simulink model "PID_LOOP"  (R2024b)
settings: Solver=FixedStepAuto  StartTime=0.0  StopTime=60  RelTol=1e-3
model workspace (MAT data in the model file):
  Drag_Constants = 1
  mass = [5.51 5.51 5.51 1 1 1]
  mass_6a = [5 5 5 1 1 1]
values from neighbouring files (symbols this model uses):
  drag_wrench = [ ... (first row only)    [constants.m]    (also in constants.mat = [0.41 0 0 0 0 0 0 0.5 0 0 0 0 ... (36 elements, 6x6)])
  g = 9.8067    [constants.m]    (also in constants.mat = 9.80665)
  I_x = 1    [constants.mat]
  I_y = 1    [constants.mat]
  I_z = 1    [constants.mat]
  m = mc + mp    (= 6)    [calculate_inertia.m]    (also in constants.mat = 5.51; mass_properties.mat = 10)
  volume = 0.0074    [constants.m]    (also in constants.mat = 0.0073741788)
  volume_center = [0, 0, -0.07]    [constants.m]    (also in constants.mat = [0 0 0.1])
  water_density = 997    [constants.m]    (also in constants.mat = 1000)
  wrench = eval(w)    [calculate_wrench.m]    (also in constants.m = geometry_properties.wrench; constants.mat = [0 0 0 0 -0.7071 -0.7071 -0.7071 -0.7071 0 0 0 0 ... (48 ele; geometry_properties.mat = [0 0 -1 0.22 0.25 0 0 0 -1 -0.22 0.25 0 ... (48 elements, 6x; wrench.m)
undefined symbols (not defined in the file or in its folder): pwm_stop
libraries: slpidlib x6, simulink x3, shareduavrstlib x1
settings Model: Creator=zenyn  LastModifiedBy=Pamarit - Test
settings DataIOCC: LoggingToFile=on
settings OptimizationCC: DefaultParameterBehavior=Inlined  UseDivisionForNetSlopeComputation=on  GainParamInheritBuiltInType=on  UseFloatMulNetSlope=on  DefaultUnderspecifiedDataType=single  InlineInvariantSignals=on  ReuseModelBlockBuffer=off  PassReuseOutputArgsAs=Individual arguments  ZeroExternalMemoryAtStartup=off  ZeroInternalMemoryAtStartup=off  NoFixptDivByZeroProtection=on  EfficientFloat2IntCast=on  LifeSpan=1  OptimizeDataStoreBuffers=off  BusAssignmentInplaceUpdate=off  EfficientTunableParamExpr=on
settings DebuggingCC: ParameterTunabilityLossMsg=error  SFUnexpectedBacktrackingDiag=warning  SFNoUnconditionalDefaultTransitionDiag=warning  UnderSpecifiedDimensionMsg=warning
settings HardwareCC: ProdLongLongMode=on
settings SFSimCC: MATLABDynamicMemAlloc=off
settings RTWCC: Description=Embedded Coder  SystemTargetFile=ert.tlc  TemplateMakefile=ert_default_tmf  GenerateReport=on  Toolchain=MinGW64 | gmake (64-bit Windows)  BuildConfiguration=Debug  IncludeHyperlinkInReport=on  LaunchReport=on  TargetLang=C++  GenerateTraceInfo=on  GenerateTraceReport=on  GenerateTraceReportSl=on  GenerateTraceReportSf=on  GenerateTraceReportEml=on
settings CodeAppCC: ForceParamTrailComments=on  IgnoreCustomStorageClasses=off  OperatorAnnotations=on  SimulinkDataObjDesc=on  SFDataObjDesc=on  CustomSymbolStrGlobalVar=rt$N$M  CustomSymbolStrType=$N$M  CustomSymbolStrFcn=$N$M$F  CustomSymbolStrMacro=$N$M  InsertBlockDesc=on  EnableCustomComments=on  ReqsInCode=on
settings ERTTargetCC: TargetLangStandard=C++11 (ISO)  GenerateSampleERTMain=on  IncludeMdlTerminateFcn=off  CombineSignalStateStructs=on  SupportAbsoluteTime=off  CodeInterfacePackaging=C++ class  SupportComplex=off  SupportContinuousTime=on  SupportNonInlinedSFcns=on  RootIOFormat=Structure reference  ERTCustomFileTemplate=example_file_process.tlc  ERTFilePackagingFormat=CompactWithDataFile  ConvertIfToSwitch=off

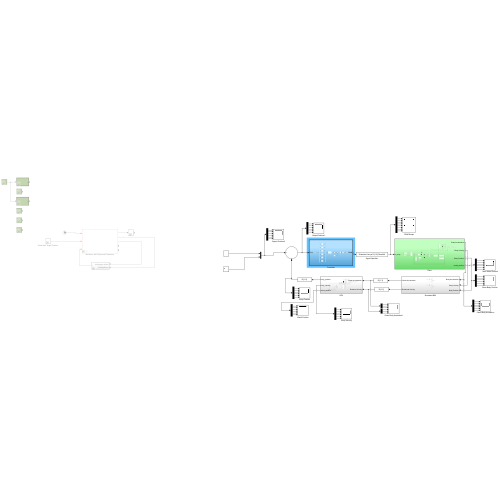
[thumbnail: Simulink's stored preview of the top-level diagram]
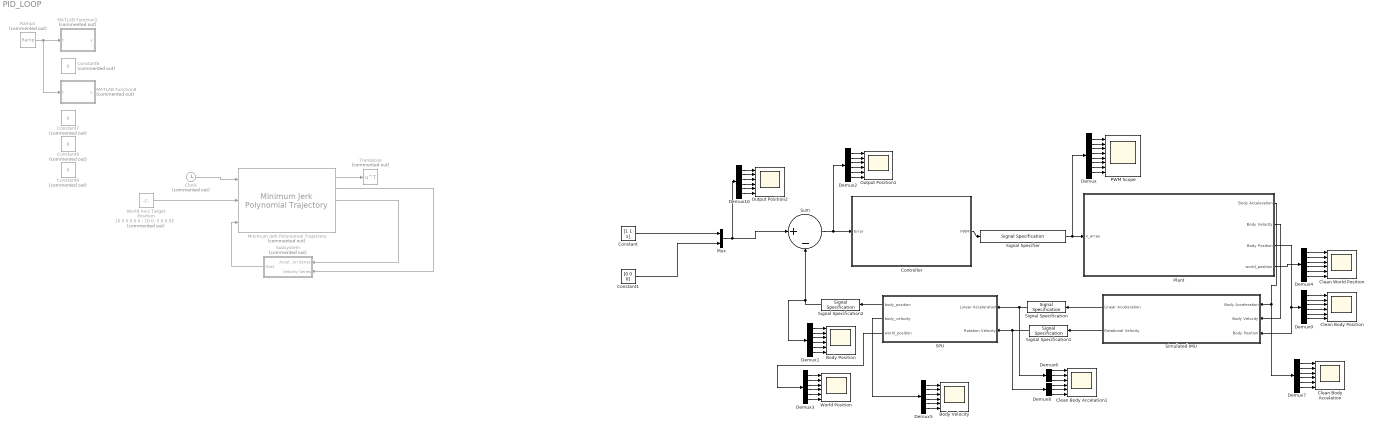
== system PID_LOOP ==
  Body Position : Scope  NumInputPorts=6
  Body Velocity : Scope  NumInputPorts=6
  Clean Body Accelation : Scope  NumInputPorts=6
  Clean Body Accelation1 : Scope  NumInputPorts=6
  Clean Body Position : Scope  NumInputPorts=6
  Clean World Position : Scope  NumInputPorts=6
  Clock : Clock  Commented=on
  Constant : Constant  Value=[1 1 1]
  Constant1 : Constant  Value=[0 0 0]
  Constant{6..9} (4 alike) : Constant  Commented=on  Value=0
  Controller : Subsystem  TreatAsAtomicUnit=on
  Demux : Demux  Outputs=8
  Demux{1..5,7,9..10} (8 alike) : Demux  Outputs=6
  Demux6 : Demux  Outputs=3
  Demux8 : Demux  Outputs=3
  MATLAB Function1 : MATLAB Function  Commented=on  TreatAsAtomicUnit=on
  MATLAB Function8 : MATLAB Function  Commented=on  TreatAsAtomicUnit=on
  Minimum Jerk Polynomial Trajectory : shareduavrstlib/Minimum Jerk Polynomial Trajectory  Commented=on  ShowBCInputPort=off  ShowPolynomialCoefs=off  ShowStatusOutputPort=off  TimeAllocation=off  TimeWeight=100  MinSegmentTime=0.1  MaxSegmentTime=1  MaxIteration=1500  MaxTime=10  SimulateUsing=Interpreted execution
      settings: LibrarySourceBlock=uavalgslib/Minimum Jerk Polynomial Trajectory
  Mux : Mux  Inputs=2
  Output Position1 : Scope  NumInputPorts=6
  Output Position2 : Scope  NumInputPorts=6
  PWM Scope : Scope  NumInputPorts=8
  Plant : Subsystem
  Ramp1 : simulink/Sources/Ramp  Commented=on  slope=1  start=0  InitialOutput=0
  SPU : Subsystem
  Signal Specification : SignalSpecification  Dimensions=[1 3]
  Signal Specification1 : SignalSpecification  Dimensions=[1 3]
  Signal Specification2 : SignalSpecification  Dimensions=[1 6]
  Signal Specifier : SignalSpecification  OutMin=[1200 ]  OutMax=[ 1800 ]  OutDataTypeStr=double  Unit=µs  Dimensions=[1 8]
  Simulated IMU : Subsystem
  Subsystem : Subsystem  Commented=on
  Sum : Sum  Inputs=|+-
  Transpose : Math  Commented=on  Operator=transpose
  World Axis Target Position : Constant  Commented=on  Value=[0 0 0 0 0 0 ; 10 0 -5 0 0 0]'
  World Position : Scope  NumInputPorts=6
  wires:
  Sum/1 -> Demux2/1, Controller/1(Error)
  Controller/1(PWM) -> Signal Specifier/1
  Ramp1/1 -> MATLAB Function8/1(t), MATLAB Function1/1(t)
  Minimum Jerk Polynomial Trajectory/1 -> Transpose/1
  Signal Specifier/1 -> Demux/1, Plant/1(x_array)
  Demux/1 -> PWM Scope/1
  Demux/2 -> PWM Scope/2
  Demux/3 -> PWM Scope/3
  Demux/4 -> PWM Scope/4
  Demux/5 -> PWM Scope/5
  Demux/6 -> PWM Scope/6
  Demux/7 -> PWM Scope/7
  Demux/8 -> PWM Scope/8
  SPU/1(body_position) -> Signal Specification2/1
  Demux1/1 -> Body Position/1
  Demux1/3 -> Body Position/3
  Demux1/6 -> Body Position/6
  Demux1/5 -> Body Position/5
  Demux1/2 -> Body Position/2
  Demux1/4 -> Body Position/4
  Demux2/1 -> Output Position1/1
  Demux2/2 -> Output Position1/2
  Demux2/3 -> Output Position1/3
  Demux2/5 -> Output Position1/5
  Demux2/6 -> Output Position1/6
  Demux2/4 -> Output Position1/4
  SPU/3(world_position) -> Demux3/1
  Demux3/3 -> World Position/3
  Demux3/4 -> World Position/4
  Demux3/6 -> World Position/6
  Demux3/2 -> World Position/2
  Demux3/1 -> World Position/1
  Demux3/5 -> World Position/5
  Demux4/1 -> Clean World Position/1
  Demux4/6 -> Clean World Position/6
  Demux4/5 -> Clean World Position/5
  Demux4/4 -> Clean World Position/4
  Demux4/3 -> Clean World Position/3
  Demux4/2 -> Clean World Position/2
  Plant/4(world_position) -> Demux4/1
  Demux5/1 -> Body Velocity/1
  Demux5/3 -> Body Velocity/3
  Demux5/2 -> Body Velocity/2
  Demux5/4 -> Body Velocity/4
  Demux5/5 -> Body Velocity/5
  Demux5/6 -> Body Velocity/6
  SPU/2(body_velocity) -> Demux5/1
  Simulated IMU/1(Linear Acceleration) -> Signal Specification/1
  Plant/1(Body Acceleration) -> Demux7/1, Simulated IMU/1(Body Acceleration)
  Demux7/1 -> Clean Body Accelation/1
  Demux7/4 -> Clean Body Accelation/4
  Demux7/5 -> Clean Body Accelation/5
  Demux7/2 -> Clean Body Accelation/2
  Demux7/6 -> Clean Body Accelation/6
  Demux7/3 -> Clean Body Accelation/3
  Plant/2(Body Velocity) -> Simulated IMU/2(Body Velocity)
  Simulated IMU/2(Rotational Velocity) -> Signal Specification1/1
  Signal Specification/1 -> Demux6/1, SPU/1(Linear Acceleration)
  Signal Specification1/1 -> Demux8/1, SPU/2(Rotation Velocity)
  Signal Specification2/1 -> Demux1/1, Sum/2
  Demux6/1 -> Clean Body Accelation1/1
  Demux6/2 -> Clean Body Accelation1/2
  Demux6/3 -> Clean Body Accelation1/3
  Demux8/1 -> Clean Body Accelation1/4
  Demux8/2 -> Clean Body Accelation1/5
  Demux8/3 -> Clean Body Accelation1/6
  Demux9/4 -> Clean Body Position/4
  Plant/3(Body Position) -> Demux9/1, Simulated IMU/3(Body Position)
  Demux9/1 -> Clean Body Position/1
  Demux9/5 -> Clean Body Position/5
  Demux9/2 -> Clean Body Position/2
  Demux9/6 -> Clean Body Position/6
  Demux9/3 -> Clean Body Position/3
  Minimum Jerk Polynomial Trajectory/2 -> Subsystem/2(Velocity Series)
  Minimum Jerk Polynomial Trajectory/3 -> Subsystem/1(Acceleration Series)
  World Axis Target Position/1 -> Minimum Jerk Polynomial Trajectory/2
  Clock/1 -> Minimum Jerk Polynomial Trajectory/1
  Demux10/4 -> Output Position2/4
  Demux10/6 -> Output Position2/6
  Demux10/5 -> Output Position2/5
  Demux10/3 -> Output Position2/3
  Demux10/2 -> Output Position2/2
  Demux10/1 -> Output Position2/1
  Subsystem/1(Out1) -> Minimum Jerk Polynomial Trajectory/3
  Constant/1 -> Mux/1
  Constant1/1 -> Mux/2
  Mux/1 -> Demux10/1, Sum/1

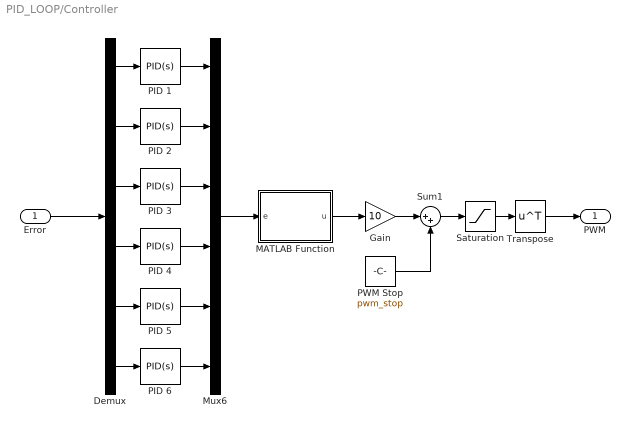
== system PID_LOOP/Controller ==
  Error : Inport
  Demux : Demux  Outputs=6
  Gain : Gain  Gain=10
  MATLAB Function : MATLAB Function  TreatAsAtomicUnit=on
  Mux6 : Mux  Inputs=6
  PID 1 : slpidlib/PID Controller  Controller=PID  Form=Parallel  TimeDomain=Continuous-time  UseExternalTs=off  SampleTime=-1  IntegratorMethod=Forward Euler  FilterMethod=Forward Euler  ControllerParametersSource=internal  P=50  I=1  UseKiTs=off  D=80  UseExternalDerivativeSource=off  N=100  UseFilter=on  TunerSelectOption=Transfer Function Based (PID Tuner App)  InitialConditionSource=internal  InitialConditionForIntegrator=0  InitialConditionForFilter=0  DifferentiatorICPrevScaledInput=0  ExternalReset=none  TrackingMode=off  Kt=1  LimitOutput=off  SatLimitsSource=internal  UpperSaturationLimit=inf  LowerSaturationLimit=-inf  LinearizeAsGain=on  AntiWindupMode=none  Kb=1  LimitIntegrator=off  UpperIntegratorSaturationLimit=inf  LowerIntegratorSaturationLimit=-inf  POutMin=[]  POutMax=[]  IOutMin=[]  IOutMax=[]  DOutMin=[]  DOutMax=[]  NOutMin=[]  NOutMax=[]  SumOutMin=[]  SumOutMax=[]  SaturationOutMin=[]  SaturationOutMax=[]  PParamMin=[]  PParamMax=[]  IParamMin=[]  IParamMax=[]  DParamMin=[]  DParamMax=[]  NParamMin=[]  NParamMax=[]  KbParamMin=[]  KbParamMax=[]  KtParamMin=[]  KtParamMax=[]  KbOutMin=[]  KbOutMax=[]  KtOutMin=[]  KtOutMax=[]  IntegratorOutMin=[]  IntegratorOutMax=[]  FilterOutMin=[]  FilterOutMax=[]  SumI1OutMin=[]  SumI1OutMax=[]  SumI2OutMin=[]  SumI2OutMax=[]  SumI3OutMin=[]  SumI3OutMax=[]  SumI4OutMin=[]  SumI4OutMax=[]  SumDOutMin=[]  SumDOutMax=[]  DifferentiatorOutMin=[]  DifferentiatorOutMax=[]  FilterDiffOutCoefMin=[]  FilterDiffOutCoefMax=[]  ReciprocalOutMin=[]  ReciprocalOutMax=[]  SumDenOutMin=[]  SumDenOutMax=[]  SumNumOutMin=[]  SumNumOutMax=[]  DivideOutMin=[]  DivideOutMax=[]  UdiffTsProdOutMin=[]  UdiffTsProdOutMax=[]  NTsProdOutMin=[]  NTsProdOutMax=[]  UintegralTsProdOutMin=[]  UintegralTsProdOutMax=[]  UngainTsProdOutMin=[]  UngainTsProdOutMax=[]  ClampingZeroOutDataTypeStr=Inherit: Inherit via back propagation  ClampingZeroOutMin=[]  ClampingZeroOutMax=[]  FilterDenConstantOutDataTypeStr=Inherit: Inherit via back propagation  FilterDenConstantOutMin=[]  FilterDenConstantOutMax=[]  PCopyOutDataTypeStr=Inherit: Inherit via back propagation  PCopyOutMin=[]  PCopyOutMax=[]  NCopyOutDataTypeStr=Inherit: Inherit via back propagation  NCopyOutMin=[]  NCopyOutMax=[]  IntegratorContinuousStateAttributes=''  IntegratorStateMustResolveToSignalObject=off  IntegratorRTWStateStorageClass=Auto  FilterContinuousStateAttributes=''  FilterStateMustResolveToSignalObject=off  FilterRTWStateStorageClass=Auto  ParallelPVariant=InternalParameters  IdealPVariant=Disabled  IVariant=InternalParameters  DVariant=InternalParameters  IntegratorVariant=Continuous  SatVariant=Disabled  AWVariant=Passthrough  PCopyVariant=Disabled  TRVariant=Disabled  FdbkBlocksVariant=Forward  IdealPFdbkVariant=Disabled  SatFdbkVariant=Disabled  DerivativeFilterVariant=ContFilter  NVariant=InternalParameters  NCopyVariant=Disabled  FilterICVariant=InternalICsFilter  IntegratorICVariant=InternalICs  ExternalResetVariant=Disabled  TRSumVariant=Passthrough  SumFdbkVariant=Disabled  SumVariant=Sum_PID  TsampFilterVariant=InternalTs  TsampNgainVariant=Passthrough  TsampIntegralVariant=Disabled_SignalSpec  ExternalSaturationOutDataTypeStr=Inherit: Same as second input  DerivativeSourceVariant=ErrorSignal  PreIntVariant=InternalPreInt
  PID 2 : slpidlib/PID Controller  Controller=PID  Form=Parallel  TimeDomain=Continuous-time  UseExternalTs=off  SampleTime=-1  IntegratorMethod=Forward Euler  FilterMethod=Forward Euler  ControllerParametersSource=internal  P=20  I=1  UseKiTs=off  D=20  UseExternalDerivativeSource=off  N=100  UseFilter=on  TunerSelectOption=Transfer Function Based (PID Tuner App)  InitialConditionSource=internal  InitialConditionForIntegrator=0  InitialConditionForFilter=0  DifferentiatorICPrevScaledInput=0  ExternalReset=none  TrackingMode=off  Kt=1  LimitOutput=off  SatLimitsSource=internal  UpperSaturationLimit=inf  LowerSaturationLimit=-inf  LinearizeAsGain=on  AntiWindupMode=none  Kb=1  LimitIntegrator=off  UpperIntegratorSaturationLimit=inf  LowerIntegratorSaturationLimit=-inf  POutMin=[]  POutMax=[]  IOutMin=[]  IOutMax=[]  DOutMin=[]  DOutMax=[]  NOutMin=[]  NOutMax=[]  SumOutMin=[]  SumOutMax=[]  SaturationOutMin=[]  SaturationOutMax=[]  PParamMin=[]  PParamMax=[]  IParamMin=[]  IParamMax=[]  DParamMin=[]  DParamMax=[]  NParamMin=[]  NParamMax=[]  KbParamMin=[]  KbParamMax=[]  KtParamMin=[]  KtParamMax=[]  KbOutMin=[]  KbOutMax=[]  KtOutMin=[]  KtOutMax=[]  IntegratorOutMin=[]  IntegratorOutMax=[]  FilterOutMin=[]  FilterOutMax=[]  SumI1OutMin=[]  SumI1OutMax=[]  SumI2OutMin=[]  SumI2OutMax=[]  SumI3OutMin=[]  SumI3OutMax=[]  SumI4OutMin=[]  SumI4OutMax=[]  SumDOutMin=[]  SumDOutMax=[]  DifferentiatorOutMin=[]  DifferentiatorOutMax=[]  FilterDiffOutCoefMin=[]  FilterDiffOutCoefMax=[]  ReciprocalOutMin=[]  ReciprocalOutMax=[]  SumDenOutMin=[]  SumDenOutMax=[]  SumNumOutMin=[]  SumNumOutMax=[]  DivideOutMin=[]  DivideOutMax=[]  UdiffTsProdOutMin=[]  UdiffTsProdOutMax=[]  NTsProdOutMin=[]  NTsProdOutMax=[]  UintegralTsProdOutMin=[]  UintegralTsProdOutMax=[]  UngainTsProdOutMin=[]  UngainTsProdOutMax=[]  ClampingZeroOutDataTypeStr=Inherit: Inherit via back propagation  ClampingZeroOutMin=[]  ClampingZeroOutMax=[]  FilterDenConstantOutDataTypeStr=Inherit: Inherit via back propagation  FilterDenConstantOutMin=[]  FilterDenConstantOutMax=[]  PCopyOutDataTypeStr=Inherit: Inherit via back propagation  PCopyOutMin=[]  PCopyOutMax=[]  NCopyOutDataTypeStr=Inherit: Inherit via back propagation  NCopyOutMin=[]  NCopyOutMax=[]  IntegratorContinuousStateAttributes=''  IntegratorStateMustResolveToSignalObject=off  IntegratorRTWStateStorageClass=Auto  FilterContinuousStateAttributes=''  FilterStateMustResolveToSignalObject=off  FilterRTWStateStorageClass=Auto  ParallelPVariant=InternalParameters  IdealPVariant=Disabled  IVariant=InternalParameters  DVariant=InternalParameters  IntegratorVariant=Continuous  SatVariant=Disabled  AWVariant=Passthrough  PCopyVariant=Disabled  TRVariant=Disabled  FdbkBlocksVariant=Forward  IdealPFdbkVariant=Disabled  SatFdbkVariant=Disabled  DerivativeFilterVariant=ContFilter  NVariant=InternalParameters  NCopyVariant=Disabled  FilterICVariant=InternalICsFilter  IntegratorICVariant=InternalICs  ExternalResetVariant=Disabled  TRSumVariant=Passthrough  SumFdbkVariant=Disabled  SumVariant=Sum_PID  TsampFilterVariant=InternalTs  TsampNgainVariant=Passthrough  TsampIntegralVariant=Disabled_SignalSpec  ExternalSaturationOutDataTypeStr=Inherit: Same as second input  DerivativeSourceVariant=ErrorSignal  PreIntVariant=InternalPreInt
  PID 3 : slpidlib/PID Controller  Controller=PID  Form=Parallel  TimeDomain=Continuous-time  UseExternalTs=off  SampleTime=-1  IntegratorMethod=Forward Euler  FilterMethod=Forward Euler  ControllerParametersSource=internal  P=40  I=1  UseKiTs=off  D=40  UseExternalDerivativeSource=off  N=100  UseFilter=on  TunerSelectOption=Transfer Function Based (PID Tuner App)  InitialConditionSource=internal  InitialConditionForIntegrator=0  InitialConditionForFilter=0  DifferentiatorICPrevScaledInput=0  ExternalReset=none  TrackingMode=off  Kt=1  LimitOutput=off  SatLimitsSource=internal  UpperSaturationLimit=inf  LowerSaturationLimit=-inf  LinearizeAsGain=on  AntiWindupMode=none  Kb=1  LimitIntegrator=off  UpperIntegratorSaturationLimit=inf  LowerIntegratorSaturationLimit=-inf  POutMin=[]  POutMax=[]  IOutMin=[]  IOutMax=[]  DOutMin=[]  DOutMax=[]  NOutMin=[]  NOutMax=[]  SumOutMin=[]  SumOutMax=[]  SaturationOutMin=[]  SaturationOutMax=[]  PParamMin=[]  PParamMax=[]  IParamMin=[]  IParamMax=[]  DParamMin=[]  DParamMax=[]  NParamMin=[]  NParamMax=[]  KbParamMin=[]  KbParamMax=[]  KtParamMin=[]  KtParamMax=[]  KbOutMin=[]  KbOutMax=[]  KtOutMin=[]  KtOutMax=[]  IntegratorOutMin=[]  IntegratorOutMax=[]  FilterOutMin=[]  FilterOutMax=[]  SumI1OutMin=[]  SumI1OutMax=[]  SumI2OutMin=[]  SumI2OutMax=[]  SumI3OutMin=[]  SumI3OutMax=[]  SumI4OutMin=[]  SumI4OutMax=[]  SumDOutMin=[]  SumDOutMax=[]  DifferentiatorOutMin=[]  DifferentiatorOutMax=[]  FilterDiffOutCoefMin=[]  FilterDiffOutCoefMax=[]  ReciprocalOutMin=[]  ReciprocalOutMax=[]  SumDenOutMin=[]  SumDenOutMax=[]  SumNumOutMin=[]  SumNumOutMax=[]  DivideOutMin=[]  DivideOutMax=[]  UdiffTsProdOutMin=[]  UdiffTsProdOutMax=[]  NTsProdOutMin=[]  NTsProdOutMax=[]  UintegralTsProdOutMin=[]  UintegralTsProdOutMax=[]  UngainTsProdOutMin=[]  UngainTsProdOutMax=[]  ClampingZeroOutDataTypeStr=Inherit: Inherit via back propagation  ClampingZeroOutMin=[]  ClampingZeroOutMax=[]  FilterDenConstantOutDataTypeStr=Inherit: Inherit via back propagation  FilterDenConstantOutMin=[]  FilterDenConstantOutMax=[]  PCopyOutDataTypeStr=Inherit: Inherit via back propagation  PCopyOutMin=[]  PCopyOutMax=[]  NCopyOutDataTypeStr=Inherit: Inherit via back propagation  NCopyOutMin=[]  NCopyOutMax=[]  IntegratorContinuousStateAttributes=''  IntegratorStateMustResolveToSignalObject=off  IntegratorRTWStateStorageClass=Auto  FilterContinuousStateAttributes=''  FilterStateMustResolveToSignalObject=off  FilterRTWStateStorageClass=Auto  ParallelPVariant=InternalParameters  IdealPVariant=Disabled  IVariant=InternalParameters  DVariant=InternalParameters  IntegratorVariant=Continuous  SatVariant=Disabled  AWVariant=Passthrough  PCopyVariant=Disabled  TRVariant=Disabled  FdbkBlocksVariant=Forward  IdealPFdbkVariant=Disabled  SatFdbkVariant=Disabled  DerivativeFilterVariant=ContFilter  NVariant=InternalParameters  NCopyVariant=Disabled  FilterICVariant=InternalICsFilter  IntegratorICVariant=InternalICs  ExternalResetVariant=Disabled  TRSumVariant=Passthrough  SumFdbkVariant=Disabled  SumVariant=Sum_PID  TsampFilterVariant=InternalTs  TsampNgainVariant=Passthrough  TsampIntegralVariant=Disabled_SignalSpec  ExternalSaturationOutDataTypeStr=Inherit: Same as second input  DerivativeSourceVariant=ErrorSignal  PreIntVariant=InternalPreInt
  PID 4 : slpidlib/PID Controller  Controller=PID  Form=Parallel  TimeDomain=Continuous-time  UseExternalTs=off  SampleTime=-1  IntegratorMethod=Forward Euler  FilterMethod=Forward Euler  ControllerParametersSource=internal  P=20  I=1  UseKiTs=off  D=20  UseExternalDerivativeSource=off  N=100  UseFilter=on  TunerSelectOption=Transfer Function Based (PID Tuner App)  InitialConditionSource=internal  InitialConditionForIntegrator=0  InitialConditionForFilter=0  DifferentiatorICPrevScaledInput=0  ExternalReset=none  TrackingMode=off  Kt=1  LimitOutput=off  SatLimitsSource=internal  UpperSaturationLimit=inf  LowerSaturationLimit=-inf  LinearizeAsGain=on  AntiWindupMode=none  Kb=1  LimitIntegrator=off  UpperIntegratorSaturationLimit=inf  LowerIntegratorSaturationLimit=-inf  POutMin=[]  POutMax=[]  IOutMin=[]  IOutMax=[]  DOutMin=[]  DOutMax=[]  NOutMin=[]  NOutMax=[]  SumOutMin=[]  SumOutMax=[]  SaturationOutMin=[]  SaturationOutMax=[]  PParamMin=[]  PParamMax=[]  IParamMin=[]  IParamMax=[]  DParamMin=[]  DParamMax=[]  NParamMin=[]  NParamMax=[]  KbParamMin=[]  KbParamMax=[]  KtParamMin=[]  KtParamMax=[]  KbOutMin=[]  KbOutMax=[]  KtOutMin=[]  KtOutMax=[]  IntegratorOutMin=[]  IntegratorOutMax=[]  FilterOutMin=[]  FilterOutMax=[]  SumI1OutMin=[]  SumI1OutMax=[]  SumI2OutMin=[]  SumI2OutMax=[]  SumI3OutMin=[]  SumI3OutMax=[]  SumI4OutMin=[]  SumI4OutMax=[]  SumDOutMin=[]  SumDOutMax=[]  DifferentiatorOutMin=[]  DifferentiatorOutMax=[]  FilterDiffOutCoefMin=[]  FilterDiffOutCoefMax=[]  ReciprocalOutMin=[]  ReciprocalOutMax=[]  SumDenOutMin=[]  SumDenOutMax=[]  SumNumOutMin=[]  SumNumOutMax=[]  DivideOutMin=[]  DivideOutMax=[]  UdiffTsProdOutMin=[]  UdiffTsProdOutMax=[]  NTsProdOutMin=[]  NTsProdOutMax=[]  UintegralTsProdOutMin=[]  UintegralTsProdOutMax=[]  UngainTsProdOutMin=[]  UngainTsProdOutMax=[]  ClampingZeroOutDataTypeStr=Inherit: Inherit via back propagation  ClampingZeroOutMin=[]  ClampingZeroOutMax=[]  FilterDenConstantOutDataTypeStr=Inherit: Inherit via back propagation  FilterDenConstantOutMin=[]  FilterDenConstantOutMax=[]  PCopyOutDataTypeStr=Inherit: Inherit via back propagation  PCopyOutMin=[]  PCopyOutMax=[]  NCopyOutDataTypeStr=Inherit: Inherit via back propagation  NCopyOutMin=[]  NCopyOutMax=[]  IntegratorContinuousStateAttributes=''  IntegratorStateMustResolveToSignalObject=off  IntegratorRTWStateStorageClass=Auto  FilterContinuousStateAttributes=''  FilterStateMustResolveToSignalObject=off  FilterRTWStateStorageClass=Auto  ParallelPVariant=InternalParameters  IdealPVariant=Disabled  IVariant=InternalParameters  DVariant=InternalParameters  IntegratorVariant=Continuous  SatVariant=Disabled  AWVariant=Passthrough  PCopyVariant=Disabled  TRVariant=Disabled  FdbkBlocksVariant=Forward  IdealPFdbkVariant=Disabled  SatFdbkVariant=Disabled  DerivativeFilterVariant=ContFilter  NVariant=InternalParameters  NCopyVariant=Disabled  FilterICVariant=InternalICsFilter  IntegratorICVariant=InternalICs  ExternalResetVariant=Disabled  TRSumVariant=Passthrough  SumFdbkVariant=Disabled  SumVariant=Sum_PID  TsampFilterVariant=InternalTs  TsampNgainVariant=Passthrough  TsampIntegralVariant=Disabled_SignalSpec  ExternalSaturationOutDataTypeStr=Inherit: Same as second input  DerivativeSourceVariant=ErrorSignal  PreIntVariant=InternalPreInt
  PID 5 : slpidlib/PID Controller  Controller=PID  Form=Parallel  TimeDomain=Continuous-time  UseExternalTs=off  SampleTime=-1  IntegratorMethod=Forward Euler  FilterMethod=Forward Euler  ControllerParametersSource=internal  P=20  I=1  UseKiTs=off  D=50  UseExternalDerivativeSource=off  N=100  UseFilter=on  TunerSelectOption=Transfer Function Based (PID Tuner App)  InitialConditionSource=internal  InitialConditionForIntegrator=0  InitialConditionForFilter=0  DifferentiatorICPrevScaledInput=0  ExternalReset=none  TrackingMode=off  Kt=1  LimitOutput=off  SatLimitsSource=internal  UpperSaturationLimit=inf  LowerSaturationLimit=-inf  LinearizeAsGain=on  AntiWindupMode=none  Kb=1  LimitIntegrator=off  UpperIntegratorSaturationLimit=inf  LowerIntegratorSaturationLimit=-inf  POutMin=[]  POutMax=[]  IOutMin=[]  IOutMax=[]  DOutMin=[]  DOutMax=[]  NOutMin=[]  NOutMax=[]  SumOutMin=[]  SumOutMax=[]  SaturationOutMin=[]  SaturationOutMax=[]  PParamMin=[]  PParamMax=[]  IParamMin=[]  IParamMax=[]  DParamMin=[]  DParamMax=[]  NParamMin=[]  NParamMax=[]  KbParamMin=[]  KbParamMax=[]  KtParamMin=[]  KtParamMax=[]  KbOutMin=[]  KbOutMax=[]  KtOutMin=[]  KtOutMax=[]  IntegratorOutMin=[]  IntegratorOutMax=[]  FilterOutMin=[]  FilterOutMax=[]  SumI1OutMin=[]  SumI1OutMax=[]  SumI2OutMin=[]  SumI2OutMax=[]  SumI3OutMin=[]  SumI3OutMax=[]  SumI4OutMin=[]  SumI4OutMax=[]  SumDOutMin=[]  SumDOutMax=[]  DifferentiatorOutMin=[]  DifferentiatorOutMax=[]  FilterDiffOutCoefMin=[]  FilterDiffOutCoefMax=[]  ReciprocalOutMin=[]  ReciprocalOutMax=[]  SumDenOutMin=[]  SumDenOutMax=[]  SumNumOutMin=[]  SumNumOutMax=[]  DivideOutMin=[]  DivideOutMax=[]  UdiffTsProdOutMin=[]  UdiffTsProdOutMax=[]  NTsProdOutMin=[]  NTsProdOutMax=[]  UintegralTsProdOutMin=[]  UintegralTsProdOutMax=[]  UngainTsProdOutMin=[]  UngainTsProdOutMax=[]  ClampingZeroOutDataTypeStr=Inherit: Inherit via back propagation  ClampingZeroOutMin=[]  ClampingZeroOutMax=[]  FilterDenConstantOutDataTypeStr=Inherit: Inherit via back propagation  FilterDenConstantOutMin=[]  FilterDenConstantOutMax=[]  PCopyOutDataTypeStr=Inherit: Inherit via back propagation  PCopyOutMin=[]  PCopyOutMax=[]  NCopyOutDataTypeStr=Inherit: Inherit via back propagation  NCopyOutMin=[]  NCopyOutMax=[]  IntegratorContinuousStateAttributes=''  IntegratorStateMustResolveToSignalObject=off  IntegratorRTWStateStorageClass=Auto  FilterContinuousStateAttributes=''  FilterStateMustResolveToSignalObject=off  FilterRTWStateStorageClass=Auto  ParallelPVariant=InternalParameters  IdealPVariant=Disabled  IVariant=InternalParameters  DVariant=InternalParameters  IntegratorVariant=Continuous  SatVariant=Disabled  AWVariant=Passthrough  PCopyVariant=Disabled  TRVariant=Disabled  FdbkBlocksVariant=Forward  IdealPFdbkVariant=Disabled  SatFdbkVariant=Disabled  DerivativeFilterVariant=ContFilter  NVariant=InternalParameters  NCopyVariant=Disabled  FilterICVariant=InternalICsFilter  IntegratorICVariant=InternalICs  ExternalResetVariant=Disabled  TRSumVariant=Passthrough  SumFdbkVariant=Disabled  SumVariant=Sum_PID  TsampFilterVariant=InternalTs  TsampNgainVariant=Passthrough  TsampIntegralVariant=Disabled_SignalSpec  ExternalSaturationOutDataTypeStr=Inherit: Same as second input  DerivativeSourceVariant=ErrorSignal  PreIntVariant=InternalPreInt
  PID 6 : slpidlib/PID Controller  Controller=PID  Form=Parallel  TimeDomain=Continuous-time  UseExternalTs=off  SampleTime=-1  IntegratorMethod=Forward Euler  FilterMethod=Forward Euler  ControllerParametersSource=internal  P=5  I=1  UseKiTs=off  D=5  UseExternalDerivativeSource=off  N=100  UseFilter=on  TunerSelectOption=Transfer Function Based (PID Tuner App)  InitialConditionSource=internal  InitialConditionForIntegrator=0  InitialConditionForFilter=0  DifferentiatorICPrevScaledInput=0  ExternalReset=none  TrackingMode=off  Kt=1  LimitOutput=off  SatLimitsSource=internal  UpperSaturationLimit=inf  LowerSaturationLimit=-inf  LinearizeAsGain=on  AntiWindupMode=none  Kb=1  LimitIntegrator=off  UpperIntegratorSaturationLimit=inf  LowerIntegratorSaturationLimit=-inf  POutMin=[]  POutMax=[]  IOutMin=[]  IOutMax=[]  DOutMin=[]  DOutMax=[]  NOutMin=[]  NOutMax=[]  SumOutMin=[]  SumOutMax=[]  SaturationOutMin=[]  SaturationOutMax=[]  PParamMin=[]  PParamMax=[]  IParamMin=[]  IParamMax=[]  DParamMin=[]  DParamMax=[]  NParamMin=[]  NParamMax=[]  KbParamMin=[]  KbParamMax=[]  KtParamMin=[]  KtParamMax=[]  KbOutMin=[]  KbOutMax=[]  KtOutMin=[]  KtOutMax=[]  IntegratorOutMin=[]  IntegratorOutMax=[]  FilterOutMin=[]  FilterOutMax=[]  SumI1OutMin=[]  SumI1OutMax=[]  SumI2OutMin=[]  SumI2OutMax=[]  SumI3OutMin=[]  SumI3OutMax=[]  SumI4OutMin=[]  SumI4OutMax=[]  SumDOutMin=[]  SumDOutMax=[]  DifferentiatorOutMin=[]  DifferentiatorOutMax=[]  FilterDiffOutCoefMin=[]  FilterDiffOutCoefMax=[]  ReciprocalOutMin=[]  ReciprocalOutMax=[]  SumDenOutMin=[]  SumDenOutMax=[]  SumNumOutMin=[]  SumNumOutMax=[]  DivideOutMin=[]  DivideOutMax=[]  UdiffTsProdOutMin=[]  UdiffTsProdOutMax=[]  NTsProdOutMin=[]  NTsProdOutMax=[]  UintegralTsProdOutMin=[]  UintegralTsProdOutMax=[]  UngainTsProdOutMin=[]  UngainTsProdOutMax=[]  ClampingZeroOutDataTypeStr=Inherit: Inherit via back propagation  ClampingZeroOutMin=[]  ClampingZeroOutMax=[]  FilterDenConstantOutDataTypeStr=Inherit: Inherit via back propagation  FilterDenConstantOutMin=[]  FilterDenConstantOutMax=[]  PCopyOutDataTypeStr=Inherit: Inherit via back propagation  PCopyOutMin=[]  PCopyOutMax=[]  NCopyOutDataTypeStr=Inherit: Inherit via back propagation  NCopyOutMin=[]  NCopyOutMax=[]  IntegratorContinuousStateAttributes=''  IntegratorStateMustResolveToSignalObject=off  IntegratorRTWStateStorageClass=Auto  FilterContinuousStateAttributes=''  FilterStateMustResolveToSignalObject=off  FilterRTWStateStorageClass=Auto  ParallelPVariant=InternalParameters  IdealPVariant=Disabled  IVariant=InternalParameters  DVariant=InternalParameters  IntegratorVariant=Continuous  SatVariant=Disabled  AWVariant=Passthrough  PCopyVariant=Disabled  TRVariant=Disabled  FdbkBlocksVariant=Forward  IdealPFdbkVariant=Disabled  SatFdbkVariant=Disabled  DerivativeFilterVariant=ContFilter  NVariant=InternalParameters  NCopyVariant=Disabled  FilterICVariant=InternalICsFilter  IntegratorICVariant=InternalICs  ExternalResetVariant=Disabled  TRSumVariant=Passthrough  SumFdbkVariant=Disabled  SumVariant=Sum_PID  TsampFilterVariant=InternalTs  TsampNgainVariant=Passthrough  TsampIntegralVariant=Disabled_SignalSpec  ExternalSaturationOutDataTypeStr=Inherit: Same as second input  DerivativeSourceVariant=ErrorSignal  PreIntVariant=InternalPreInt
  PWM Stop : Constant  Value=pwm_stop
  Saturation : Saturate  UpperLimit=1900  LowerLimit=1100
  Sum1 : Sum  Inputs=|++
  Transpose : Math  Operator=transpose
  PWM : Outport
  wires:
  Error/1 -> Demux/1
  PWM Stop/1 -> Sum1/2
  Mux6/1 -> MATLAB Function/1(e)
  MATLAB Function/1(u) -> Gain/1
  Gain/1 -> Sum1/1
  Sum1/1 -> Saturation/1
  Saturation/1 -> Transpose/1
  Transpose/1 -> PWM/1
  Demux/6 -> PID 6/1
  Demux/5 -> PID 5/1
  Demux/4 -> PID 4/1
  Demux/3 -> PID 3/1
  Demux/2 -> PID 2/1
  Demux/1 -> PID 1/1
  PID 1/1 -> Mux6/1
  PID 2/1 -> Mux6/2
  PID 3/1 -> Mux6/3
  PID 4/1 -> Mux6/4
  PID 5/1 -> Mux6/5
  PID 6/1 -> Mux6/6

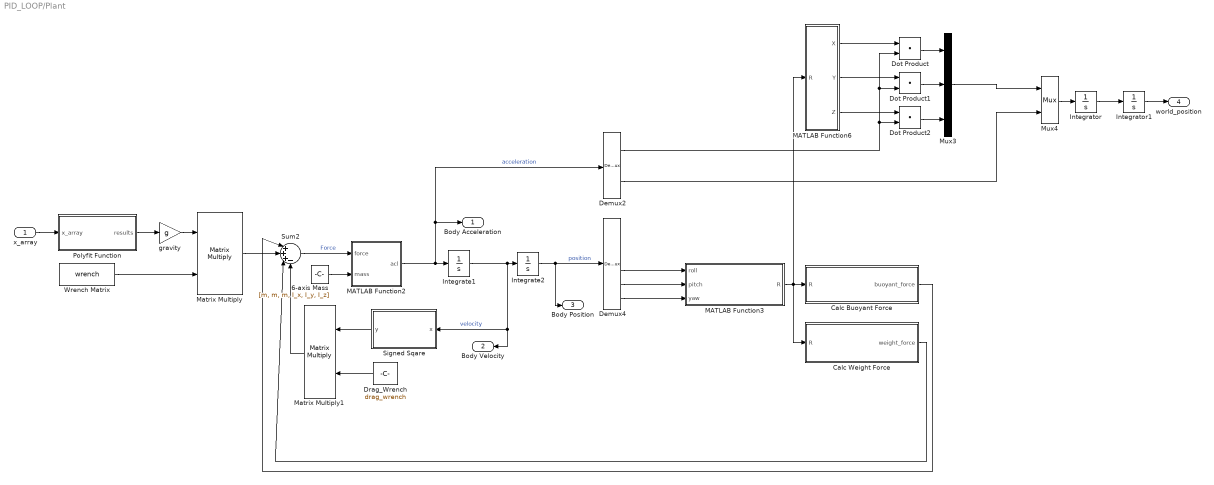
== system PID_LOOP/Plant ==
  x_array : Inport
  6-axis Mass : Constant  Value=[m, m, m, I_x, I_y, I_z]  VectorParams1D=off
  Calc Buoyant Force : MATLAB Function  TreatAsAtomicUnit=on
  Calc Weight Force : MATLAB Function  TreatAsAtomicUnit=on
  Demux2 : Demux  Outputs=2
  Demux4 : Demux  Outputs=6
  Dot Product : DotProduct  OutDataTypeStr=Inherit: Inherit via internal rule
  Dot Product1 : DotProduct  OutDataTypeStr=Inherit: Inherit via internal rule
  Dot Product2 : DotProduct  OutDataTypeStr=Inherit: Inherit via internal rule
  Drag_Wrench : Constant  Value=drag_wrench  VectorParams1D=off
  Integrate1 : Integrator
  Integrate2 : Integrator
  Integrator : Integrator
  Integrator1 : Integrator
  MATLAB Function2 : MATLAB Function  TreatAsAtomicUnit=on
  MATLAB Function3 : MATLAB Function  TreatAsAtomicUnit=on
  MATLAB Function6 : MATLAB Function  TreatAsAtomicUnit=on
  Matrix Multiply : Product  Multiplication=Matrix(*)
  Matrix Multiply1 : Product  Multiplication=Matrix(*)
  Mux3 : Mux  Inputs=3
  Mux4 : Mux  Inputs=2
  Polyfit Function : MATLAB Function  TreatAsAtomicUnit=on
  Signed Sqare : MATLAB Function  TreatAsAtomicUnit=on
  Sum2 : Sum  Inputs=|+++-
  Wrench Matrix : Constant  Value=wrench  VectorParams1D=off
  gravity : Gain  Gain=g
  Body Acceleration : Outport
  Body Velocity : Outport  Port=2
  Body Position : Outport  Port=3
  world_position : Outport  Port=4
  wires:
  Demux4/5 -> MATLAB Function3/2(pitch)
  Matrix Multiply/1 -> Sum2/2
  Integrate2/1 -> Body Position/1, Demux4/1  "position"
  x_array/1 -> Polyfit Function/1(x_array)
  Signed Sqare/1(y) -> Matrix Multiply1/1
  MATLAB Function3/1(R) -> Calc Weight Force/1(R), Calc Buoyant Force/1(R), MATLAB Function6/1(R)
  Sum2/1 -> MATLAB Function2/1(force)  "Force"
  Drag_Wrench/1 -> Matrix Multiply1/2
  Calc Weight Force/1(weight_force) -> Sum2/3
  Demux4/6 -> MATLAB Function3/3(yaw)
  gravity/1 -> Matrix Multiply/1
  Polyfit Function/1(results) -> gravity/1
  Demux4/4 -> MATLAB Function3/1(roll)
  Wrench Matrix/1 -> Matrix Multiply/2
  Integrate1/1 -> Integrate2/1, Body Velocity/1, Signed Sqare/1(x)  "velocity"
  Matrix Multiply1/1 -> Sum2/4
  Calc Buoyant Force/1(buoyant_force) -> Sum2/1
  MATLAB Function2/1(acl) -> Demux2/1, Body Acceleration/1, Integrate1/1  "acceleration"
  6-axis Mass/1 -> MATLAB Function2/2(mass)
  Mux3/1 -> Mux4/1
  MATLAB Function6/2(Y) -> Dot Product1/1
  Dot Product/1 -> Mux3/1
  Demux2/1 -> Dot Product2/2, Dot Product1/2, Dot Product/2
  Dot Product1/1 -> Mux3/2
  MATLAB Function6/1(X) -> Dot Product/1
  Integrator1/1 -> world_position/1
  Mux4/1 -> Integrator/1
  Integrator/1 -> Integrator1/1
  Dot Product2/1 -> Mux3/3
  MATLAB Function6/3(Z) -> Dot Product2/1
  Demux2/2 -> Mux4/2

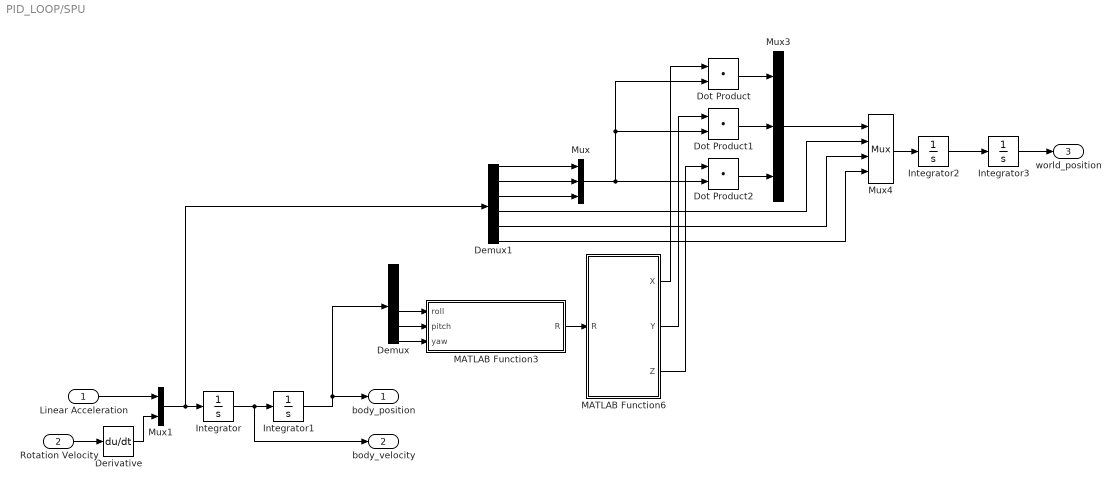
== system PID_LOOP/SPU ==
  Linear Acceleration : Inport
  Rotation Velocity : Inport  Port=2
  Demux : Demux  Outputs=6
  Demux1 : Demux  Outputs=6
  Derivative : Derivative
  Dot Product : DotProduct  OutDataTypeStr=Inherit: Inherit via internal rule
  Dot Product1 : DotProduct  OutDataTypeStr=Inherit: Inherit via internal rule
  Dot Product2 : DotProduct  OutDataTypeStr=Inherit: Inherit via internal rule
  Integrator{,1..3} (4 alike) : Integrator
  MATLAB Function3 : MATLAB Function  TreatAsAtomicUnit=on
  MATLAB Function6 : MATLAB Function  TreatAsAtomicUnit=on
  Mux : Mux  Inputs=3
  Mux1 : Mux  Inputs=2
  Mux3 : Mux  Inputs=3
  Mux4 : Mux
  body_position : Outport
  body_velocity : Outport  Port=2
  world_position : Outport  Port=3
  wires:
  Integrator1/1 -> Demux/1, body_position/1
  Dot Product1/1 -> Mux3/2
  Dot Product2/1 -> Mux3/3
  MATLAB Function6/3(Z) -> Dot Product2/1
  Mux3/1 -> Mux4/1
  Integrator3/1 -> world_position/1
  Integrator2/1 -> Integrator3/1
  MATLAB Function6/2(Y) -> Dot Product1/1
  Mux4/1 -> Integrator2/1
  MATLAB Function6/1(X) -> Dot Product/1
  Dot Product/1 -> Mux3/1
  Demux/4 -> MATLAB Function3/1(roll)
  Demux/5 -> MATLAB Function3/2(pitch)
  Demux/6 -> MATLAB Function3/3(yaw)
  MATLAB Function3/1(R) -> MATLAB Function6/1(R)
  Demux1/4 -> Mux4/2
  Demux1/5 -> Mux4/3
  Demux1/6 -> Mux4/4
  Demux1/1 -> Mux/1
  Demux1/2 -> Mux/2
  Demux1/3 -> Mux/3
  Mux/1 -> Dot Product/2, Dot Product1/2, Dot Product2/2
  Rotation Velocity/1 -> Derivative/1
  Linear Acceleration/1 -> Mux1/1
  Mux1/1 -> Demux1/1, Integrator/1
  Integrator/1 -> body_velocity/1, Integrator1/1
  Derivative/1 -> Mux1/2

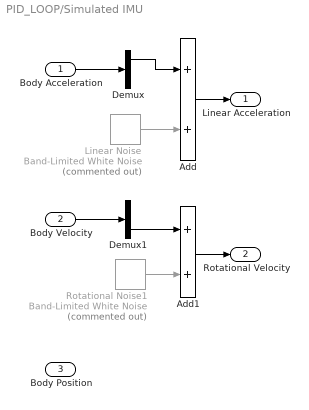
== system PID_LOOP/Simulated IMU ==
  Body Acceleration : Inport
  Body Velocity : Inport  Port=2
  Body Position : Inport  Port=3
  Add : Sum
  Add1 : Sum
  Demux : Demux  Outputs=2
  Demux1 : Demux  Outputs=2
  Linear Noise : simulink/Sources/Band-Limited White Noise  Commented=on  Cov=lin_noise  Ts=0.1  seed=[23341]
  Rotational Noise1 : simulink/Sources/Band-Limited White Noise  Commented=on  Cov=rot_noise  Ts=0.1  seed=[23341]
  Linear Acceleration : Outport
  Rotational Velocity : Outport  Port=2
  wires:
  Add/1 -> Linear Acceleration/1
  Add1/1 -> Rotational Velocity/1
  Body Acceleration/1 -> Demux/1
  Demux/1 -> Add/1
  Linear Noise/1 -> Add/2
  Rotational Noise1/1 -> Add1/2
  Body Velocity/1 -> Demux1/1
  Demux1/2 -> Add1/1

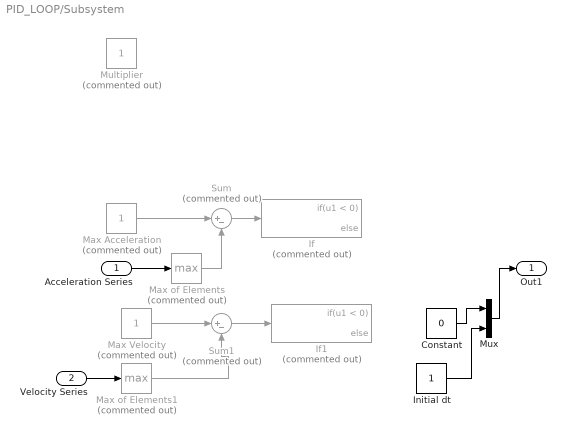
== system PID_LOOP/Subsystem ==
  Acceleration Series : Inport
  Velocity Series : Inport  Port=2
  Constant : Constant  Value=0
  If : If  Commented=on  IfExpression=u1 < 0
  If1 : If  Commented=on  IfExpression=u1 < 0
  Initial dt : Constant
  Max Acceleration : Constant  Commented=on
  Max Velocity : Constant  Commented=on
  Max of Elements : MinMax  Commented=on  Function=max
  Max of Elements1 : MinMax  Commented=on  Function=max
  Multiplier : Constant  Commented=on
  Mux : Mux  Inputs=2
  Sum : Sum  Commented=on  Inputs=|+-
  Sum1 : Sum  Commented=on  Inputs=|+-
  Out1 : Outport
  wires:
  Velocity Series/1 -> Max of Elements1/1
  Acceleration Series/1 -> Max of Elements/1
  Max Acceleration/1 -> Sum/1
  Max Velocity/1 -> Sum1/1
  Sum1/1 -> If1/1
  Sum/1 -> If/1
  Max of Elements/1 -> Sum/2
  Max of Elements1/1 -> Sum1/2
  Mux/1 -> Out1/1
  Constant/1 -> Mux/1
  Initial dt/1 -> Mux/2

== matlab function PID_LOOP/MATLAB Function8 ==
  data: t input; y output
function y = fcn(t)

speed = 30 / 30; 
if t < 30
    y = 0;
elseif t < 60
    y = 30 * speed - t * speed;
else
    y = 30 * speed - 60 * speed;
end

== matlab function PID_LOOP/Plant/Signed Sqare ==
  data: x input; y output
function y = signed_square(x)
y = x .* abs(x);
end

== matlab function PID_LOOP/Plant/Polyfit Function ==
  data: x_array input; results output
function results = pwm_function(x_array)
    % this fucntion is terriblly written due to ai conversion. rewrite
    % Preallocate results array
    results = zeros(size(x_array)); 
    
    % First condition: 1100 <= x < 1460
    idx = (x_array >= 1100 & x_array < 1460);
    results(idx) = (-1.24422882971549e-8) * x_array(idx).^3 ...
                 + (4.02057100632393e-5) * x_array(idx).^2 ...
                 - 0.0348619861030835 * x_array(idx) ...
                 + 3.90671429105423;
    
    % Second condition: 1460 <= x <= 1540
    idx = (x_array >= 1460 & x_array <= 1540);
    results(idx) = 0;
    
    % Third condition: 1540 < x <= 1900
    idx = (x_array > 1540 & x_array <= 1900);
    results(idx) = (-1.64293565374284e-8) * x_array(idx).^3 ...
                 + (9.45962838560648e-5) * x_array(idx).^2 ...
                 - 0.170812079190679 * x_array(idx) ...
                 + 98.7232373648272;
    
    % Handle out-of-range values
    if any(isnan(results))
        error('Some values in x_array are out of the valid range [1100..1900].');
    end
end

== matlab function PID_LOOP/Plant/MATLAB Function2 ==
  data: force input; acl output; mass input
function acl = fcn(force, mass)
acl = force ./ mass;

end

== matlab function PID_LOOP/Plant/MATLAB Function3 ==
  data: roll input; R output; pitch input; yaw input
function R = rotation_matrix(roll, pitch, yaw)
    % Rotation matrix around X-axis (roll)
    Rx = [
        1,  0,           0;
        0,  cos(roll),  -sin(roll);
        0,  sin(roll),   cos(roll)
    ];

    % Rotation matrix around Y-axis (pitch)
    Ry = [
        cos(pitch),  0,  sin(pitch);
        0,           1,  0;
       -sin(pitch),  0,  cos(pitch)
    ];

    % Rotation matrix around Z-axis (yaw)
    Rz = [
        cos(yaw), -sin(yaw),  0;
        sin(yaw),  cos(yaw),  0;
        0,         0,         1
    ];

    % Combine rotations: R = Rz * Ry * Rx
    R = Rz * Ry * Rx;
end

== matlab function PID_LOOP/Plant/Calc Buoyant Force ==
  data: R input; buoyant_force output; g parameter; water_density parameter; volume parameter; volume_center parameter
function buoyant_force = buoyant_force(R, g, water_density, volume, volume_center)

    % Ensure d is a column vector
    volume_center = volume_center(:);

    % Buoyant force vector in world frame
    b_vector = [0; 0; water_density * -g * volume];

    % Rotate buoyant force to object's frame
    buoyant_force_body = R * b_vector;

    % Compute torque using cross product τ = d × F_buoyancy
    % (MATLAB cross function works for column vectors)
    torque = cross(-volume_center, buoyant_force_body);

    % Combine force and torque into a single output vector
    buoyant_force = [buoyant_force_body; torque]';
end

== matlab function PID_LOOP/Plant/Calc Weight Force ==
  data: R input; weight_force output; g parameter; m parameter
function weight_force = weight_force(R, g, m)

    % Gravity force vector in world frame (downward)
    g_vector = [0; 0; m * g];
    
    % Linear Force
    lin = R * g_vector;
    % Rotational force
    rot = [0;0;0];
    % Transform gravity force to rotated frame
    weight_force = [lin', rot'];
end

== matlab function PID_LOOP/Plant/MATLAB Function6 ==
  data: R input; X output; Y output; Z output
function [X, Y, Z] =  axes(R)
% in this function, x, y and z axes refer to direction relative current
% orientation of robot

% X, Y and Z axes refer to direction relative to intial orientation of
% robot

x_vector = [1; 0; 0];
y_vector = [0; 1; 0];
z_vector = [0; 0; 1];

X = [R * x_vector];
Y = [R * y_vector];
Z = [R * z_vector];

end

== matlab function PID_LOOP/Controller/MATLAB Function ==
  data: e input; u output; wrench parameter
function u = rev_wrench(e, wrench)

inv_wrench = pinv(wrench);
u = inv_wrench' * e;

end

== matlab function PID_LOOP/MATLAB Function1 ==
  data: t input; y output
function y = fcn(t)

if t < 30
    y = t;
elseif t < 60
    y = 30;
else
    y = 90 - t;

end

== matlab function PID_LOOP/SPU/MATLAB Function6 ==
  data: R input; X output; Y output; Z output
function [X, Y, Z] =  axes(R)
% in this function, x, y and z axes refer to direction relative current
% orientation of robot

% X, Y and Z axes refer to direction relative to intial orientation of
% robot

x_vector = [1; 0; 0];
y_vector = [0; 1; 0];
z_vector = [0; 0; 1];

X = [R * x_vector];
Y = [R * y_vector];
Z = [R * z_vector];

end

== matlab function PID_LOOP/SPU/MATLAB Function3 ==
  data: roll input; R output; pitch input; yaw input
function R = rotation_matrix(roll, pitch, yaw)
    % Rotation matrix around X-axis (roll)
    Rx = [
        1,  0,           0;
        0,  cos(roll),  -sin(roll);
        0,  sin(roll),   cos(roll)
    ];

    % Rotation matrix around Y-axis (pitch)
    Ry = [
        cos(pitch),  0,  sin(pitch);
        0,           1,  0;
       -sin(pitch),  0,  cos(pitch)
    ];

    % Rotation matrix around Z-axis (yaw)
    Rz = [
        cos(yaw), -sin(yaw),  0;
        sin(yaw),  cos(yaw),  0;
        0,         0,         1
    ];

    % Combine rotations: R = Rz * Ry * Rx
    R = Rz * Ry * Rx;
end
